simulink model "Duffing"  (R2014b)
settings: Solver=ode45  StartTime=0.0  StopTime=10.0  RelTol=1e-3
values from neighbouring files (symbols this model uses):
  b = 0.7    [Run_Aizawa.m]    (also in Run_Arneodo.m = 3.5; Run_Chen.m = 3; Run_Chua.m = 28; Run_Duffing.m = 100)
  s = 3.5    [Run_Aizawa.m]    (also in Run_Chua_4D.m = 0.75; Run_Duffing.m = 0.2; Run_HindmarshRose.m = 4; Run_Lorenz.m = 10)
  w = 1    [Run_Duffing.m]
  y = 1    [Run_Duffing.m]    (also in Run_MackeyGlass.m)
undefined symbols (not defined in the file or in its folder): param
settings Model: Creator=Arek  LastModifiedBy=Arek

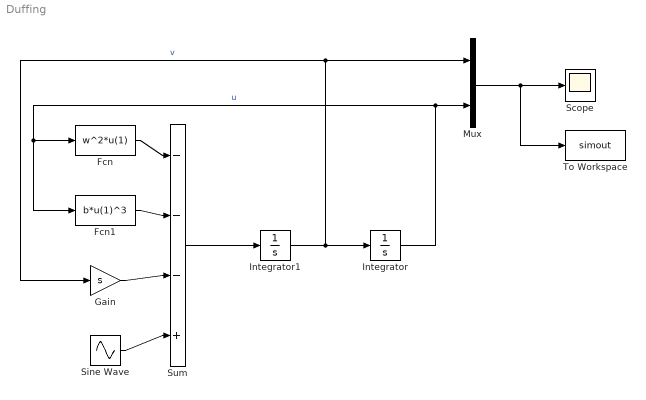
== system Duffing ==
  Fcn : Fcn  Expr=w^2*u(1)
  Fcn1 : Fcn  Expr=b*u(1)^3
  Gain : Gain  Gain=s
  Integrator : Integrator  InitialCondition=param.ic(2)
  Integrator1 : Integrator  InitialCondition=param.ic(1)
  Mux : Mux  Inputs=2
  Scope : Scope
      settings: ShowLegends=on
  Sine Wave : Sin  Amplitude=y  Frequency=w  Phase=fi  SampleTime=0
  Sum : Sum  Inputs=-|-|-|+
  To Workspace : ToWorkspace  VariableName=simout  SaveFormat=Timeseries  SampleTime=-1
  wires:
  Integrator1/1 -> Integrator/1, Mux/1, Gain/1  "v"
  Sum/1 -> Integrator1/1
  Fcn/1 -> Sum/1
  Integrator/1 -> Fcn/1, Fcn1/1, Mux/2  "u"
  Fcn1/1 -> Sum/2
  Gain/1 -> Sum/3
  Sine Wave/1 -> Sum/4
  Mux/1 -> To Workspace/1, Scope/1
